simulink model "simu2"  (R2015b)
settings: Solver=ode45  SolverMode=SingleTasking  StartTime=0.0  StopTime=35  RelTol=1e-3
undefined symbols (not defined in the file or in its folder): Am, As, Bm, Bs, Gamma1, Gamma2
settings Model: Creator=e1302259  LastModifiedBy=Kais_Mesfioui
settings DataIOCC: SaveFormat=Array
settings OptimizationCC: BlockReduction=off  BooleanDataType=off
settings DebuggingCC: SaveWithParameterizedLinksMsg=none  UnderspecifiedInitializationDetection=Classic  MergeDetectMultiDrivingBlocksExec=none  SignalResolutionControl=TryResolveAllWithWarning
settings HardwareCC: ProdBitPerPointer=32  ProdLargestAtomicFloat=None  ProdIntDivRoundTo=Undefined  ProdEndianess=Unspecified  ProdWordSize=32  ProdHWDeviceType=32-bit Generic  TargetUnknown=on
settings GRTTargetCC: GeneratePreprocessorConditionals=Disable all
settings ConfigComp: CovModelRefEnable=Off  CovSFcnEnable=off

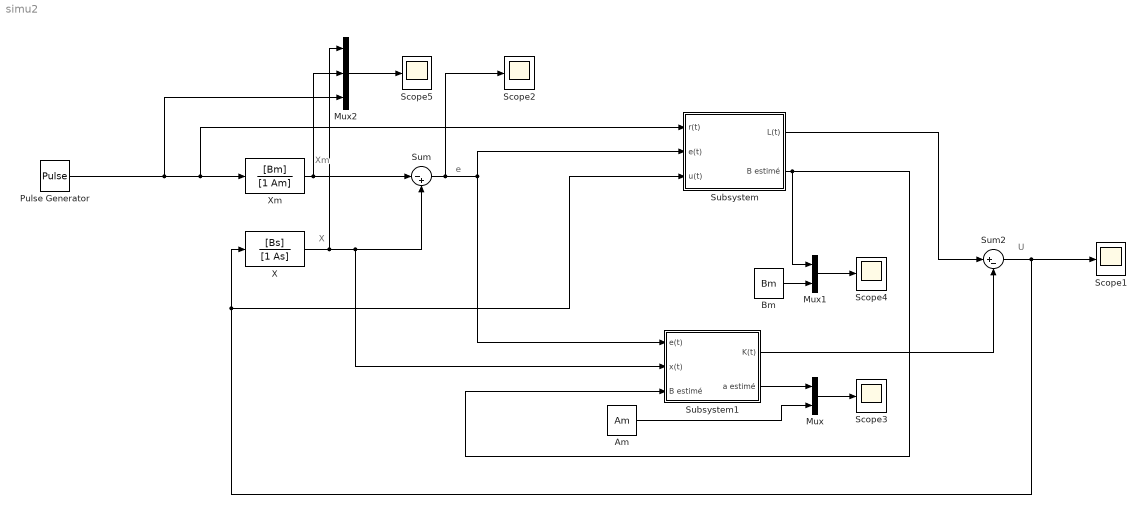
== system simu2 ==
  note: U
  note: e
  note: X
  note: Xm
  "Am " : Constant  Value=Am
  Bm : Constant  Value=Bm
  Mux : Mux  Inputs=2
  Mux1 : Mux  Inputs=2
  Mux2 : Mux  Inputs=3
  Pulse Generator : DiscretePulseGenerator  PulseType=Time based  Period=20  PulseWidth=50
  Scope{1..5} (5 alike) : Scope
  Subsystem : Subsystem
  Subsystem1 : Subsystem
  Sum : Sum  Inputs=|-+
  Sum2 : Sum  Inputs=|+-
  X : TransferFcn  Numerator=[Bs]  Denominator=[1 As]
  Xm : TransferFcn  Numerator=[Bm]  Denominator=[1 Am]
  wires:
  Xm/1 -> Mux2/2, Sum/1
  Sum/1 -> Scope2/1, Subsystem1/1(e(t)), Subsystem/2(e(t))
  X/1 -> Mux2/1, Subsystem1/2(x(t)), Sum/2
  Pulse Generator/1 -> Mux2/3, Subsystem/1(r(t)), Xm/1
  Sum2/1 -> X/1, Subsystem/3(u(t)), Scope1/1
  Subsystem/1(L(t)) -> Sum2/1
  Subsystem/2(B estimé) -> Mux1/1, Subsystem1/3(B estimé)
  Subsystem1/1(K(t)) -> Sum2/2
  Subsystem1/2(a estimé) -> Mux/1
  "Am "/1 -> Mux/2
  Mux/1 -> Scope3/1
  Bm/1 -> Mux1/2
  Mux1/1 -> Scope4/1
  Mux2/1 -> Scope5/1

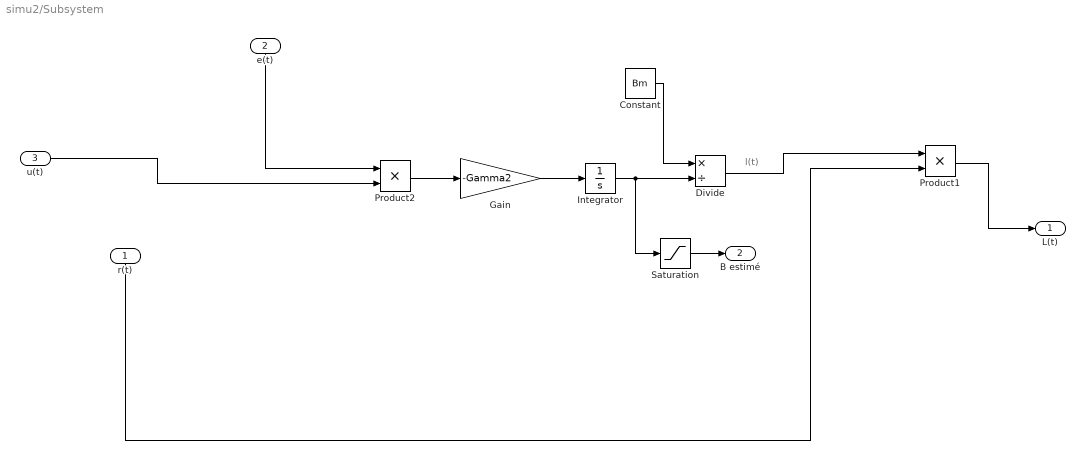
== system simu2/Subsystem ==
  note: l(t)
  r(t) : Inport
  e(t) : Inport  Port=2
  u(t) : Inport  Port=3
  Constant : Constant  Value=Bm
  Divide : Product  Inputs=*/
  Gain : Gain  Gain=-Gamma2
  Integrator : Integrator  InitialCondition=5
  Product1 : Product
  Product2 : Product
  Saturation : Saturate  UpperLimit=inf  LowerLimit=0.1
  L(t) : Outport
  B estimé : Outport  Port=2
  wires:
  Product2/1 -> Gain/1
  Gain/1 -> Integrator/1
  e(t)/1 -> Product2/1
  u(t)/1 -> Product2/2
  r(t)/1 -> Product1/2
  Integrator/1 -> Saturation/1, Divide/2
  Divide/1 -> Product1/1
  Product1/1 -> L(t)/1
  Constant/1 -> Divide/1
  Saturation/1 -> B estimé/1

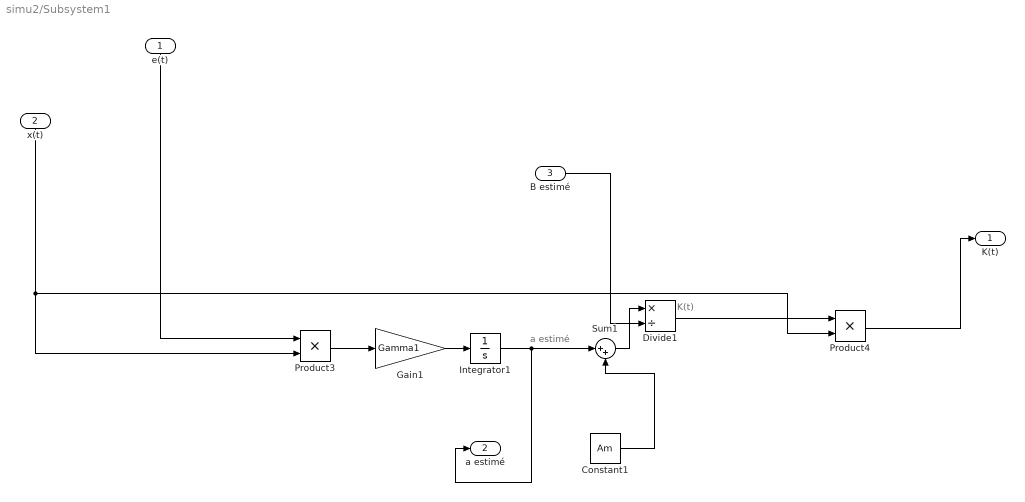
== system simu2/Subsystem1 ==
  note: K(t)
  note: a estimé
  e(t) : Inport
  x(t) : Inport  Port=2
  B estimé : Inport  Port=3
  Constant1 : Constant  Value=Am
  Divide1 : Product  Inputs=*/
  Gain1 : Gain  Gain=Gamma1
  Integrator1 : Integrator  InitialCondition=5
  Product3 : Product
  Product4 : Product
  Sum1 : Sum  Inputs=|++
  K(t) : Outport
  a estimé : Outport  Port=2
  wires:
  Product3/1 -> Gain1/1
  Gain1/1 -> Integrator1/1
  Constant1/1 -> Sum1/2
  Product4/1 -> K(t)/1
  B estimé/1 -> Divide1/2
  e(t)/1 -> Product3/1
  x(t)/1 -> Product4/2, Product3/2
  Divide1/1 -> Product4/1
  Sum1/1 -> Divide1/1
  Integrator1/1 -> a estimé/1, Sum1/1
